simulink model "UAV_Task4_3"  (R2024b)
settings: Solver=ode45  StartTime=0  StopTime=100  RelTol=1e-5  AbsTol=1e-5
values from neighbouring files (symbols this model uses):
  adaptiveActivation = 1    [UAV_Task4_1_main.m]    (also in UAV_Task4_2_main.m = 0; UAV_Task4_3_main.m)
  B_p = 1/UAV.m    [UAV_Task4_1_main.m]    (also in UAV_Task4_2_main.m; UAV_Task4_3_main.m)
  F2plus = F2'*pinv(F2*F2')    [UAV_Task4_1_main.m]    (also in UAV_Task4_2_main.m; UAV_Task4_3_main.m)
  fe_0 = [0;0]    [UAV_Task4_3_main.m]
  Gamma_a = 1*[1 1 1 1]'    [UAV_Task4_1_main.m]    (also in UAV_Task4_2_main.m; UAV_Task4_3_main.m = 1*[1 1 1 1 1 1]')
  Gamma_a_scalar = 1    [UAV_Task4_2_main.m]    (also in UAV_Task4_3_main.m)
  gravityInAdaptiveController = 1    [UAV_Task4_1_main.m]    (also in UAV_Task4_2_main.m; UAV_Task4_3_main.m)
  k_f = 0.3379e-6    (= 3.379e-07)    [UAV_Task4_1_main.m]    (also in UAV_Task4_2_main.m; UAV_Task4_3_main.m)
  L = 10    [UAV_Task4_1_main.m]    (also in UAV_Task4_2_main.m; UAV_Task4_3_main.m)
  lambda_0 = 1    [UAV_Task4_1_main.m]    (also in UAV_Task4_2_main.m; UAV_Task4_3_main.m)
  Omega_0 = [1500 1500 1500 1500]'    [UAV_Task4_1_main.m]    (also in UAV_Task4_2_main.m; UAV_Task4_3_main.m)
  omegab_0 = [0; 0; 0]    [UAV_Task4_1_main.m]    (also in UAV_Task4_2_main.m; UAV_Task4_3_main.m)
  p_0 = [0; 0; 0]    [UAV_Task4_1_main.m]    (also in UAV_Task4_2_main.m; UAV_Task4_3_main.m)
  PO = 1    [UAV_Task4_1_main.m]    (also in UAV_Task4_2_main.m; UAV_Task4_3_main.m)
  q_0 = eul2quat([0, 0, 0]*degToRad,'ZYX')'    [UAV_Task4_1_main.m]    (also in UAV_Task4_2_main.m; UAV_Task4_3_main.m)
  scenario = 2    [UAV_Task4_1_main.m]    (also in UAV_Task4_2_main.m; UAV_Task4_3_main.m)
  theta_0 = [0.07;0.07;0.1]    [UAV_Task4_1_main.m]    (also in UAV_Task4_2_main.m; UAV_Task4_3_main.m)
  vb_0 = [0; 0; 0]    [UAV_Task4_1_main.m]    (also in UAV_Task4_2_main.m; UAV_Task4_3_main.m)
undefined symbols (not defined in the file or in its folder): adaptive_controller, ctrl, D_fv_i, dyn, e_3, epsilon_PO, fw_params_fc, g, lambda_i, par, pos, pos_pp, projection_operator, targetParams, theta_M, UAV, v_M, vel, vel_pp
libraries: slpidlib x22, matrix_library x6, aerolibutil x2, uavutilslib x1
(part 1 of 4)
settings Model: Creator=justs  LastModifiedBy=giuseppe
settings SolverCC: ZeroCrossAlgorithm=Adaptive
settings DataIOCC: SaveFormat=StructureWithTime
settings OptimizationCC: BlockReduction=off  BufferReuse=off  ReuseModelBlockBuffer=off
settings DebuggingCC: AlgebraicLoopMsg=none
settings ModelReferenceCC: EnableRefExpFcnMdlSchedulingChecks=on
settings RTWCC: GPUComputeCapability=3.5

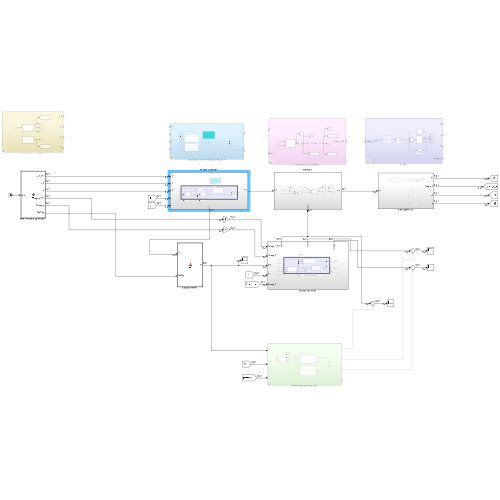
[thumbnail: Simulink's stored preview of the top-level diagram]
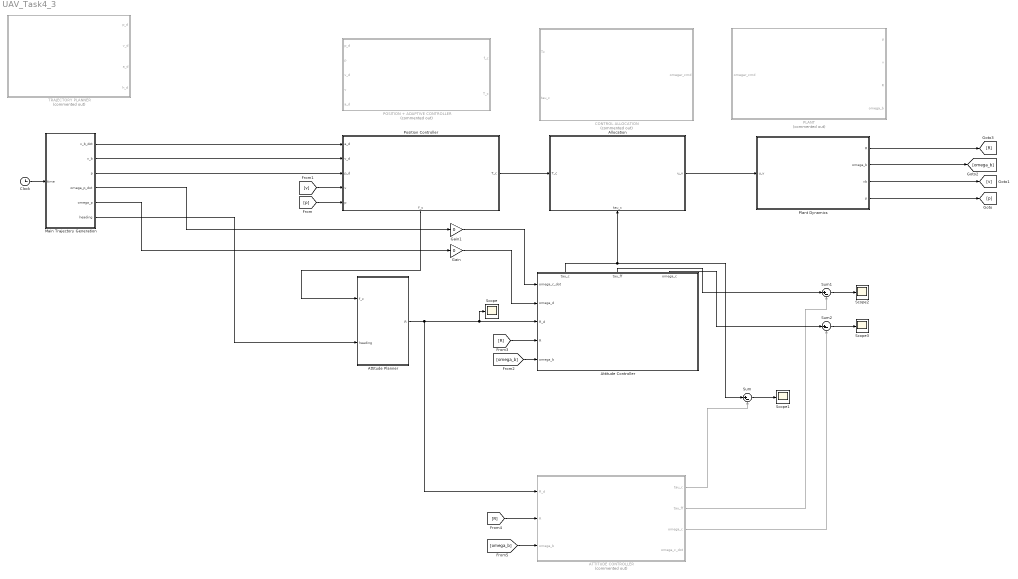
== system UAV_Task4_3 ==
  ATTITUDE CONTROLLER : Subsystem  Commented=on
  Allocation : Subsystem
      settings: PortSchema="{\"entries\":[{\"content\":{\"sides\":[{\"content\":{\"connectorIds\":[\"In1\"]},\"type\":\"ConnectorPlacement.EquallySpacedRectSide\",\"uuid\":\"a90dffa2-e17d-417b-aee2-5b49e390cc31\"},{\"content\":{\"connectorIds\":[\"Out1\"],\"side\":\"RIGHT\"},\"type\":\"ConnectorPlacement.EquallySpacedRectSide\",\"uuid\":\"68e70ff2-14f1-48b3-bfaa-1f22ab14f6ef\"},{\"content\":{\"side\":\"TOP\"},\"type\":\"ConnectorPlacement.EquallySpacedRectSide\",\"uuid\":\"a590dd5a-1e20-4e52-b823-4efe502fedb5\"},{\"content\":{\"connectorIds\":[\"In2\"],\"side\":\"BOTTOM\"},\"type\":\"ConnectorPlacement.EquallySpacedRectSide\",\"uuid\":\"c0eee0c2-1b4f-48e1-a09d-5bd9eaf490e9\"}]},\"type\":\"ConnectorPlacement.EquallySpacedConnector\",\"uuid\":\"29ee6c53-58dc-46de-8e17-ce1d472e0644\"}],\"packageUris\":[\"http://schema.mathworks.com/mf0/Connector/R2020b\"],\"version\":\"1.0\"}"
  Attitude Controller : Subsystem
      settings: PortSchema="{\"entries\":[{\"content\":{\"sides\":[{\"content\":{\"connectorIds\":[\"In1\",\"In2\",\"In3\",\"In4\",\"In5\"]},\"type\":\"ConnectorPlacement.EquallySpacedRectSide\",\"uuid\":\"fd474fdd-809e-484b-b672-45c162405a48\"},{\"content\":{\"side\":\"RIGHT\"},\"type\":\"ConnectorPlacement.EquallySpacedRectSide\",\"uuid\":\"9c86daaf-9aed-46d9-83bf-dcd411d29638\"},{\"content\":{\"connectorIds\":[\"Out1\",\"Out2\",\"Out3\"],\"side\":\"TOP\"},\"type\":\"ConnectorPlacement.EquallySpacedRectSide\",\"uuid\":\"8bdcf73f-78a3-4153-a3ad-0cecea352ffe\"}]},\"type\":\"ConnectorPlacement.EquallySpacedConnector\",\"uuid\":\"4a1693e7-34c2-4f2b-859c-49762a9733c3\"}],\"packageUris\":[\"http://schema.mathworks.com/mf0/Connector/R2020b\"],\"version\":\"1.0\"}"
  Attitude Planner : MATLAB Function  TreatAsAtomicUnit=on
  CONTROL ALLOCATION : Subsystem  Commented=on
  Clock : Clock
  Gain : Gain  Gain=0
  Gain1 : Gain  Gain=0
  Main Trajectory Generation : MATLAB Function  TreatAsAtomicUnit=on
  PLANT : Subsystem  Commented=on
  POSITION + ADAPTIVE CONTROLLER : Subsystem  Commented=on
  Plant Dynamics : Subsystem
  Position Controller : Subsystem
      settings: PortSchema="{\"entries\":[{\"content\":{\"sides\":[{\"content\":{\"connectorIds\":[\"In1\",\"In2\",\"In3\",\"In4\",\"In5\"]},\"type\":\"ConnectorPlacement.EquallySpacedRectSide\",\"uuid\":\"aaf371c6-7de6-4752-a94f-8f5eebff8076\"},{\"content\":{\"connectorIds\":[\"Out1\"],\"side\":\"RIGHT\"},\"type\":\"ConnectorPlacement.EquallySpacedRectSide\",\"uuid\":\"c91caa52-c2d3-4ced-bf24-c82d170a1382\"},{\"content\":{\"side\":\"TOP\"},\"type\":\"ConnectorPlacement.EquallySpacedRectSide\",\"uuid\":\"213f93cc-3232-43d4-924b-d32a630f7005\"},{\"content\":{\"connectorIds\":[\"Out2\"],\"side\":\"BOTTOM\"},\"type\":\"ConnectorPlacement.EquallySpacedRectSide\",\"uuid\":\"34712f80-774f-4a90-8ba5-2e5f701bc3fc\"}]},\"type\":\"ConnectorPlacement.EquallySpacedConnector\",\"uuid\":\"ff6af449-8110-47b4-88e9-388be9daf96b\"}],\"packageUris\":[\"http://schema.mathworks.com/mf0/Connector/R2020b\"],\"version\":\"1.0\"}"
  Scope{,1..3} (4 alike) : Scope
  Sum : Sum  Inputs=|+-
  Sum1 : Sum  Inputs=|+-
  Sum2 : Sum  Inputs=|+-
  TRAJECTORY PLANNER : Subsystem  Commented=on
  wires:
  Allocation/1(u_v) -> Plant Dynamics/1(u_v)
  Main Trajectory Generation/4(omega_p_dot) -> Gain1/1
  Main Trajectory Generation/5(omega_p) -> Gain/1
  Main Trajectory Generation/6(heading) -> Attitude Planner/2(heading)
  Position Controller/1(T_c) -> Allocation/1(T_c)
  [omega_b] -> Attitude Controller/5(omega_b)
  [R] -> Attitude Controller/4(R)
  Attitude Planner/1(R) -> ATTITUDE CONTROLLER/1(R_d), Attitude Controller/3(R_d), Scope/1
  Position Controller/2(f_c) -> Attitude Planner/1(f_c)
  [p] -> Position Controller/5(p)
  [v] -> Position Controller/4(v)
  Plant Dynamics/1(R) -> [R]
  Plant Dynamics/2(omega_b) -> [omega_b]
  Plant Dynamics/3(vb) -> [v]
  Plant Dynamics/4(p) -> [p]
  ATTITUDE CONTROLLER/1(tau_c) -> Sum/2
  Sum/1 -> Scope1/1
  Attitude Controller/1(tau_c) -> Allocation/2(tau_c), Sum/1
  [R] -> ATTITUDE CONTROLLER/2(R)
  [omega_b] -> ATTITUDE CONTROLLER/3(omega_b)
  Clock/1 -> Main Trajectory Generation/1(time)
  Main Trajectory Generation/3(p) -> Position Controller/3(p_d)
  Main Trajectory Generation/2(v_b) -> Position Controller/2(v_d)
  Main Trajectory Generation/1(v_b_dot) -> Position Controller/1(a_d)
  Sum1/1 -> Scope2/1
  Sum2/1 -> Scope3/1
  Attitude Controller/2(tau_ff) -> Sum1/1
  ATTITUDE CONTROLLER/2(tau_ff) -> Sum1/2
  ATTITUDE CONTROLLER/3(omega_c) -> Sum2/2
  Attitude Controller/3(omega_c) -> Sum2/1
  Gain/1 -> Attitude Controller/2(omega_d)
  Gain1/1 -> Attitude Controller/1(omega_c_dot)

== system UAV_Task4_3/ATTITUDE CONTROLLER ==
  R_d : Inport
  R : Inport  Port=2
  omega_b : Inport  Port=3
  Attitude dynamics FB : Subsystem
  Attitude dynamics FF : Subsystem
  Attitude kinematics : Subsystem
  Scope : Scope
  To Workspace : ToWorkspace  Commented=on  VariableName=tau_c  SaveFormat=Structure With Time  SampleTime=-1
  tau_c : Outport
  tau_ff : Outport  Port=2
  omega_c : Outport  Port=3
  omega_c_dot : Outport  Port=4
  wires:
  R_d/1 -> Attitude kinematics/1(R_d)
  Attitude kinematics/1(omega_c) -> omega_c/1, Scope/1, [omega_c]
  Attitude kinematics/2(omega_c_dot) -> omega_c_dot/1, [omega_c_dot]
  [omega_c] -> Attitude dynamics FF/1(omega_c)
  [omega_c_dot] -> Attitude dynamics FF/2(omega_c_dot)
  omega_b/1 -> Attitude dynamics FB/1(omega_b), Attitude dynamics FF/3(omega_b)
  R/1 -> Attitude kinematics/2(R)
  [omega_c] -> Attitude dynamics FB/2(omega_c)
  Attitude dynamics FF/1(tau_c) -> To Workspace/1, tau_c/1
  Attitude dynamics FF/2(tau_ff) -> tau_ff/1

== system UAV_Task4_3/Allocation ==
  T_c : Inport
  tau_c : Inport  Port=2
  Constant : Constant  Value=F2plus
  Matrix Multiply : Product  Multiplication=Matrix(*)
  Mux2 : Mux  Inputs=2
  Reshape : Reshape  OutputDimensionality=Column vector (2-D)
  Saturation : Saturate  Commented=through  UpperLimit=1000  LowerLimit=0
  Scope : Scope
  Scope1 : Scope
  Scope2 : Scope
  u_v : Outport
  wires:
  Mux2/1 -> Reshape/1
  tau_c/1 -> Mux2/2
  Reshape/1 -> Matrix Multiply/2
  Constant/1 -> Matrix Multiply/1
  Matrix Multiply/1 -> Scope1/1, Saturation/1  "u_v"
  T_c/1 -> Mux2/1, Scope/1
  Saturation/1 -> Scope2/1, u_v/1

== system UAV_Task4_3/Attitude Controller ==
  note: Attitude Controller
  omega_c_dot : Inport
  omega_d : Inport  Port=2
  R_d : Inport  Port=3
  R : Inport  Port=4
  omega_b : Inport  Port=5
  Attitude controller (Kin) : MATLAB Function  TreatAsAtomicUnit=on
  Attitude feedforward : MATLAB Function  TreatAsAtomicUnit=on
  Derivative : Derivative
  Feedback (Angular Velocity controller) (Dyn) : Subsystem
  Sum : Sum  Inputs=+-|
  Sum1 : Sum  Inputs=|-+
  To Workspace : ToWorkspace  VariableName=e_omega  SaveFormat=Timeseries  SampleTime=-1
  To Workspace1 : ToWorkspace  VariableName=tau_c  SaveFormat=Timeseries  SampleTime=-1
  To Workspace3 : ToWorkspace  VariableName=quat_e  SaveFormat=Timeseries  SampleTime=-1
  tau_c : Outport
  tau_ff : Outport  Port=2
  omega_c : Outport  Port=3
  wires:
  R/1 -> Attitude controller (Kin)/3(R)
  R_d/1 -> Attitude controller (Kin)/1(R_d)
  Attitude controller (Kin)/2(quat_e) -> To Workspace3/1
  Sum1/1 -> Feedback (Angular Velocity controller) (Dyn)/1(e_omega), To Workspace/1
  Feedback (Angular Velocity controller) (Dyn)/1(tau_fbk) -> Sum/2
  omega_b/1 -> Attitude feedforward/1(omega_b), Sum1/2
  omega_d/1 -> Attitude controller (Kin)/2(omega_d)
  Sum/1 -> tau_c/1, To Workspace1/1  "tau_c"
  Attitude feedforward/1(tau_ff) -> tau_ff/1, Sum/1
  Attitude controller (Kin)/1(omega_c) -> Derivative/1, omega_c/1, Attitude feedforward/3(omega_c), Sum1/1
  Derivative/1 -> Attitude feedforward/2(omega_c_dot)

== system UAV_Task4_3/CONTROL ALLOCATION ==
  Tc : Inport
  tau_c : Inport  Port=2
  Gain : Gain  Commented=through  Gain=1/k_f
  MATLAB Function1 : MATLAB Function  TreatAsAtomicUnit=on
  Saturation : Saturate  UpperLimit=3  LowerLimit=0.1
  Scope : Scope
  Scope1 : Scope
  Scope2 : Scope
  Sqrt : Sqrt  Commented=through
  To Workspace : ToWorkspace  VariableName=u_c  SaveFormat=Structure With Time  SampleTime=-1
  To Workspace1 : ToWorkspace  VariableName=omegar_cmd  SaveFormat=Timeseries  SampleTime=-1
  To Workspace2 : ToWorkspace  VariableName=omegar_cmd_array  SampleTime=-1
  omegar_cmd : Outport
  wires:
  Tc/1 -> MATLAB Function1/1(Tc)
  tau_c/1 -> MATLAB Function1/2(tau_c)
  Sqrt/1 -> To Workspace1/1, Scope2/1, To Workspace2/1, omegar_cmd/1
  MATLAB Function1/1(u_c) -> Saturation/1, Scope/1
  Saturation/1 -> Gain/1, Scope1/1, To Workspace/1
  Gain/1 -> Sqrt/1

== system UAV_Task4_3/PLANT ==
  note: w_g
  note: F*u
  note: Control wrench
  note: Damping wrench
  omegar_cmd : Inport
  Add : Sum  Inputs=++-
  Gain1 : Gain  Gain=UAV.F  Multiplication=Matrix(K*u)
  Gain2 : Gain  Gain=UAV.D  Multiplication=Matrix(K*u)
  Gravity wrench : MATLAB Function  TreatAsAtomicUnit=on
  Propeller dynamics : Subsystem  Commented=through
  "Rigid Body dynamics&kinematics " : Subsystem
  p : Outport
  v : Outport  Port=2
  R : Outport  Port=3
  omega_b : Outport  Port=4
  wires:
  "Rigid Body dynamics&kinematics "/5(nu_b) -> Gain2/1
  Gravity wrench/1(w_g) -> Add/1
  Add/1 -> "Rigid Body dynamics&kinematics "/1(w_b)
  "Rigid Body dynamics&kinematics "/2(R) -> Gravity wrench/1(R), R/1
  omegar_cmd/1 -> Propeller dynamics/1(omegar_cmd)
  Propeller dynamics/1(u) -> Gain1/1
  "Rigid Body dynamics&kinematics "/1(p) -> p/1
  Gain2/1 -> Add/3  "D*nu_b"
  "Rigid Body dynamics&kinematics "/4(omegab) -> omega_b/1
  "Rigid Body dynamics&kinematics "/3(vb) -> v/1
  Gain1/1 -> Add/2

== system UAV_Task4_3/POSITION + ADAPTIVE CONTROLLER ==
  p_d : Inport
  p : Inport  Port=2
  v_d : Inport  Port=3
  v : Inport  Port=4
  a_d : Inport  Port=5
  Constant1 : Constant  Value=adaptive_controller
  MATLAB Function : MATLAB Function  TreatAsAtomicUnit=on
  P/P PARALLEL CONTROLLER : Subsystem  Commented=on
  POSITION CONTROLLER : Subsystem
  Scope : Scope
  Scope1 : Scope
  Scope5 : Scope
  Subsystem1 : Subsystem
  Sum : Sum  Inputs=|+-
  Sum1 : Sum  Inputs=++|
  Switch1 : Switch  Criteria=u2 > Threshold  Threshold=0.5  SaturateOnIntegerOverflow=off  InputSameDT=off
  To Workspace : ToWorkspace  VariableName=f_c  SaveFormat=Structure With Time  SampleTime=-1
  To Workspace1 : ToWorkspace  VariableName=T_c  SaveFormat=Structure With Time  SampleTime=-1
  To Workspace2 : ToWorkspace  VariableName=p_error  SaveFormat=Timeseries  SampleTime=-1
  f_c : Outport
  T_c : Outport  Port=2
  wires:
  p_d/1 -> Sum/1, P/P PARALLEL CONTROLLER/1(p_d), POSITION CONTROLLER/1(p_d)
  p/1 -> Sum/2, P/P PARALLEL CONTROLLER/2(p), POSITION CONTROLLER/2(p)
  v_d/1 -> P/P PARALLEL CONTROLLER/3(v_d), POSITION CONTROLLER/3(v_d)
  v/1 -> Subsystem1/1(v), P/P PARALLEL CONTROLLER/4(v), POSITION CONTROLLER/4(v)
  MATLAB Function/1(T_c) -> To Workspace1/1, T_c/1
  Switch1/1 -> MATLAB Function/1(f_c), f_c/1, Scope/1, To Workspace/1
  Sum/1 -> Scope1/1, To Workspace2/1
  Sum1/1 -> Switch1/1, Scope5/1
  Constant1/1 -> Switch1/2
  POSITION CONTROLLER/1(f_c) -> Subsystem1/2(ub), Sum1/2, Switch1/3
  a_d/1 -> P/P PARALLEL CONTROLLER/5(a_d), POSITION CONTROLLER/5(a_d)
  Subsystem1/1(ua) -> Sum1/1

== system UAV_Task4_3/Plant Dynamics ==
  note: fix UAV.F and put it here
  note: Damping wrench
  note: F*u
  note: w_g
  u_v : Inport
  Add : Sum  Commented=on  Inputs=++-
  Attitude kinematics&dynamics : Subsystem
  Gain1 : Gain  Gain=UAV.F  Multiplication=Matrix(K*u)
  Gain2 : Gain  Commented=on  Gain=UAV.D  Multiplication=Matrix(K*u)
  Gravity wrench : MATLAB Function  Commented=on  TreatAsAtomicUnit=on
  "Rigid Body dynamics&kinematics " : Subsystem  Commented=on
  Rotor Dynamics : Subsystem
  R : Outport
  omega_b : Outport  Port=2
  vb : Outport  Port=3
  p : Outport  Port=4
  wires:
  u_v/1 -> Rotor Dynamics/1(T_cmd)
  Gain2/1 -> Add/3  "D*nu_b"
  "Rigid Body dynamics&kinematics "/5(nu_b) -> Gain2/1
  "Rigid Body dynamics&kinematics "/2(R) -> Gravity wrench/1(R)
  Gravity wrench/1(w_g) -> Add/1
  Add/1 -> "Rigid Body dynamics&kinematics "/1(w_b)
  Attitude kinematics&dynamics/1(p) -> p/1
  Attitude kinematics&dynamics/2(v_NED) -> vb/1
  Attitude kinematics&dynamics/3(omega_b) -> omega_b/1
  Attitude kinematics&dynamics/4(R) -> R/1
  Rotor Dynamics/1(Actual Thrust) -> Gain1/1
  Gain1/1 -> Attitude kinematics&dynamics/1(w_b)

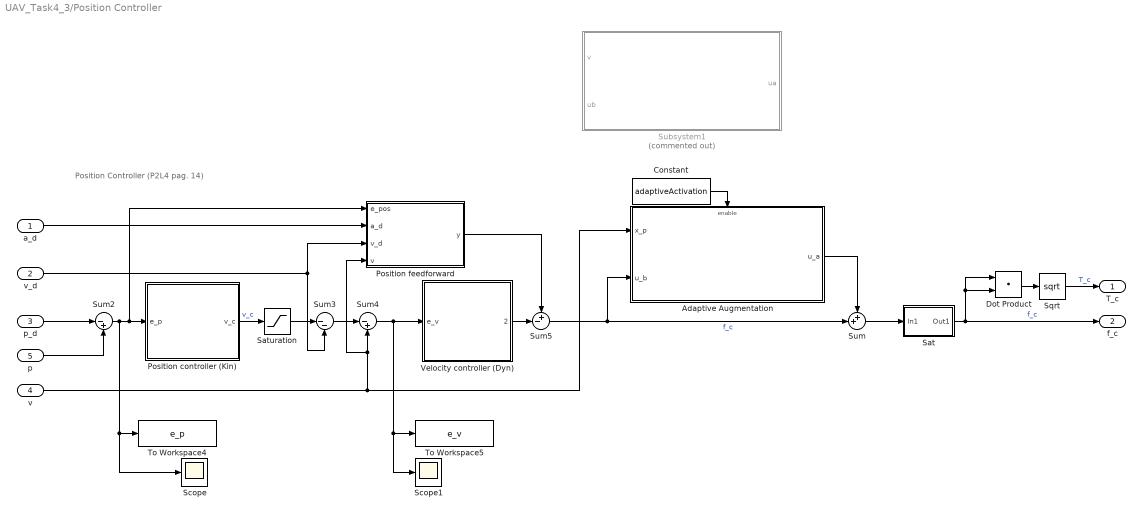
== system UAV_Task4_3/Position Controller ==
  note: Position Controller (P2L4 pag. 14)
  a_d : Inport
  v_d : Inport  Port=2
  p_d : Inport  Port=3
  v : Inport  Port=4
  p : Inport  Port=5
  Adaptive Augmentation : Subsystem
  Constant : Constant  Value=adaptiveActivation
  Dot Product : DotProduct  OutDataTypeStr=Inherit: Inherit via internal rule
  Position controller (Kin) : Subsystem
  Position feedforward : MATLAB Function  TreatAsAtomicUnit=on
  Sat : Subsystem
  Saturation : Saturate  UpperLimit=ctrl.vMax  LowerLimit=-ctrl.vMax
  Scope : Scope
  Scope1 : Scope
  Sqrt : Sqrt
  Subsystem1 : Subsystem  Commented=on
  Sum : Sum  Inputs=++|
  Sum2 : Sum  Inputs=|-+
  Sum3 : Sum  Inputs=|--
  Sum4 : Sum  Inputs=|-+
  Sum5 : Sum  Inputs=+-|
  To Workspace4 : ToWorkspace  VariableName=e_p  SaveFormat=Timeseries  SampleTime=-1
  To Workspace5 : ToWorkspace  VariableName=e_v  SaveFormat=Timeseries  SampleTime=-1
  Velocity controller (Dyn) : Subsystem
  T_c : Outport
  f_c : Outport  Port=2
  wires:
  p/1 -> Sum2/2
  a_d/1 -> Position feedforward/2(a_d)
  Sum4/1 -> Scope1/1, To Workspace5/1, Velocity controller (Dyn)/1(e_v)
  v_d/1 -> Sum3/2, Position feedforward/3(v_d)
  v/1 -> Adaptive Augmentation/1(x_p), Position feedforward/4(v), Sum4/2
  p_d/1 -> Sum2/1
  Velocity controller (Dyn)/1(2) -> Sum5/2
  Sum3/1 -> Sum4/1
  Sum2/1 -> Position feedforward/1(e_pos), Position controller (Kin)/1(e_p), Scope/1, To Workspace4/1
  Sum5/1 -> Adaptive Augmentation/2(u_b), Sum/2  "f_c"
  Position feedforward/1(y) -> Sum5/1
  Dot Product/1 -> Sqrt/1
  Sqrt/1 -> T_c/1  "T_c"
  Position controller (Kin)/1(v_c) -> Saturation/1  "v_c"
  Saturation/1 -> Sum3/1
  Sat/1(Out1) -> f_c/1, Dot Product/2, Dot Product/1  "f_c"
  Constant/1 -> Adaptive Augmentation/Enable
  Sum/1 -> Sat/1(In1)
  Adaptive Augmentation/1(u_a) -> Sum/1

== system UAV_Task4_3/TRAJECTORY PLANNER ==
  Clock : Clock
  Heading : MATLAB Function  TreatAsAtomicUnit=on
  To Workspace : ToWorkspace  VariableName=h_d  SaveFormat=Structure With Time  SampleTime=-1
  To Workspace1 : ToWorkspace  VariableName=p_d_array  SampleTime=-1
  Trajectory planner : MATLAB Function  TreatAsAtomicUnit=on
  p_d : Outport
  v_d : Outport  Port=2
  a_d : Outport  Port=3
  h_d : Outport  Port=4
  wires:
  Clock/1 -> Trajectory planner/1(t)
  Trajectory planner/3(a_d) -> a_d/1
  Trajectory planner/1(p_d) -> To Workspace1/1, p_d/1
  Trajectory planner/2(v_d) -> v_d/1
  Heading/1(h_d) -> h_d/1, To Workspace/1

== system UAV_Task4_3/ATTITUDE CONTROLLER/Attitude dynamics FB ==
  omega_b : Inport
  omega_c : Inport  Port=2
  Demux : Demux  Outputs=3
  Mux : Mux  Inputs=3
  PID Controller : slpidlib/PID Controller  Controller=PI  Form=Parallel  TimeDomain=Continuous-time  UseExternalTs=off  SampleTime=-1  IntegratorMethod=Forward Euler  FilterMethod=Forward Euler  ControllerParametersSource=internal  P=dyn.Kp(1,1)  I=dyn.Ki(1,1)  UseKiTs=off  D=dyn.Kd(1,1)  UseExternalDerivativeSource=off  N=100  UseFilter=on  TunerSelectOption=Transfer Function Based (PID Tuner App)  InitialConditionSource=internal  InitialConditionForIntegrator=0  InitialConditionForFilter=0  DifferentiatorICPrevScaledInput=0  ExternalReset=none  TrackingMode=off  Kt=1  LimitOutput=off  SatLimitsSource=internal  UpperSaturationLimit=inf  LowerSaturationLimit=-inf  LinearizeAsGain=on  AntiWindupMode=none  Kb=1  LimitIntegrator=off  UpperIntegratorSaturationLimit=inf  LowerIntegratorSaturationLimit=-inf  POutMin=[]  POutMax=[]  IOutMin=[]  IOutMax=[]  DOutMin=[]  DOutMax=[]  NOutMin=[]  NOutMax=[]  SumOutMin=[]  SumOutMax=[]  SaturationOutMin=[]  SaturationOutMax=[]  PParamMin=[]  PParamMax=[]  IParamMin=[]  IParamMax=[]  DParamMin=[]  DParamMax=[]  NParamMin=[]  NParamMax=[]  KbParamMin=[]  KbParamMax=[]  KtParamMin=[]  KtParamMax=[]  KbOutMin=[]  KbOutMax=[]  KtOutMin=[]  KtOutMax=[]  IntegratorOutMin=[]  IntegratorOutMax=[]  FilterOutMin=[]  FilterOutMax=[]  SumI1OutMin=[]  SumI1OutMax=[]  SumI2OutMin=[]  SumI2OutMax=[]  SumI3OutMin=[]  SumI3OutMax=[]  SumI4OutMin=[]  SumI4OutMax=[]  SumDOutMin=[]  SumDOutMax=[]  DifferentiatorOutMin=[]  DifferentiatorOutMax=[]  FilterDiffOutCoefMin=[]  FilterDiffOutCoefMax=[]  ReciprocalOutMin=[]  ReciprocalOutMax=[]  SumDenOutMin=[]  SumDenOutMax=[]  SumNumOutMin=[]  SumNumOutMax=[]  DivideOutMin=[]  DivideOutMax=[]  UdiffTsProdOutMin=[]  UdiffTsProdOutMax=[]  NTsProdOutMin=[]  NTsProdOutMax=[]  UintegralTsProdOutMin=[]  UintegralTsProdOutMax=[]  UngainTsProdOutMin=[]  UngainTsProdOutMax=[]  ClampingZeroOutDataTypeStr=Inherit: Inherit via back propagation  ClampingZeroOutMin=[]  ClampingZeroOutMax=[]  FilterDenConstantOutDataTypeStr=Inherit: Inherit via back propagation  FilterDenConstantOutMin=[]  FilterDenConstantOutMax=[]  PCopyOutDataTypeStr=Inherit: Inherit via back propagation  PCopyOutMin=[]  PCopyOutMax=[]  NCopyOutDataTypeStr=Inherit: Inherit via back propagation  NCopyOutMin=[]  NCopyOutMax=[]  IntegratorContinuousStateAttributes=''  IntegratorStateMustResolveToSignalObject=off  IntegratorRTWStateStorageClass=Auto  FilterContinuousStateAttributes=''  FilterStateMustResolveToSignalObject=off  FilterRTWStateStorageClass=Auto  ParallelPVariant=InternalParameters  IdealPVariant=Disabled  IVariant=InternalParameters  DVariant=Disabled  IntegratorVariant=Continuous  SatVariant=Disabled  AWVariant=Passthrough  PCopyVariant=Disabled  TRVariant=Disabled  FdbkBlocksVariant=Forward  IdealPFdbkVariant=Disabled  SatFdbkVariant=Disabled  DerivativeFilterVariant=Disabled  NVariant=Disabled  NCopyVariant=Disabled_SignalSpec  FilterICVariant=Disabled  IntegratorICVariant=InternalICs  ExternalResetVariant=Disabled  TRSumVariant=Passthrough  SumFdbkVariant=Disabled  SumVariant=Sum_PI  TsampFilterVariant=InternalTs  TsampNgainVariant=Passthrough  TsampIntegralVariant=Disabled_SignalSpec  ExternalSaturationOutDataTypeStr=Inherit: Same as second input  DerivativeSourceVariant=Disabled  PreIntVariant=InternalPreInt
  PID Controller1 : slpidlib/PID Controller  Controller=PI  Form=Parallel  TimeDomain=Continuous-time  UseExternalTs=off  SampleTime=-1  IntegratorMethod=Forward Euler  FilterMethod=Forward Euler  ControllerParametersSource=internal  P=dyn.Kp(2,2)  I=dyn.Ki(2,2)  UseKiTs=off  D=dyn.Kd(2,2)  UseExternalDerivativeSource=off  N=100  UseFilter=on  TunerSelectOption=Transfer Function Based (PID Tuner App)  InitialConditionSource=internal  InitialConditionForIntegrator=0  InitialConditionForFilter=0  DifferentiatorICPrevScaledInput=0  ExternalReset=none  TrackingMode=off  Kt=1  LimitOutput=off  SatLimitsSource=internal  UpperSaturationLimit=inf  LowerSaturationLimit=-inf  LinearizeAsGain=on  AntiWindupMode=none  Kb=1  LimitIntegrator=off  UpperIntegratorSaturationLimit=inf  LowerIntegratorSaturationLimit=-inf  POutMin=[]  POutMax=[]  IOutMin=[]  IOutMax=[]  DOutMin=[]  DOutMax=[]  NOutMin=[]  NOutMax=[]  SumOutMin=[]  SumOutMax=[]  SaturationOutMin=[]  SaturationOutMax=[]  PParamMin=[]  PParamMax=[]  IParamMin=[]  IParamMax=[]  DParamMin=[]  DParamMax=[]  NParamMin=[]  NParamMax=[]  KbParamMin=[]  KbParamMax=[]  KtParamMin=[]  KtParamMax=[]  KbOutMin=[]  KbOutMax=[]  KtOutMin=[]  KtOutMax=[]  IntegratorOutMin=[]  IntegratorOutMax=[]  FilterOutMin=[]  FilterOutMax=[]  SumI1OutMin=[]  SumI1OutMax=[]  SumI2OutMin=[]  SumI2OutMax=[]  SumI3OutMin=[]  SumI3OutMax=[]  SumI4OutMin=[]  SumI4OutMax=[]  SumDOutMin=[]  SumDOutMax=[]  DifferentiatorOutMin=[]  DifferentiatorOutMax=[]  FilterDiffOutCoefMin=[]  FilterDiffOutCoefMax=[]  ReciprocalOutMin=[]  ReciprocalOutMax=[]  SumDenOutMin=[]  SumDenOutMax=[]  SumNumOutMin=[]  SumNumOutMax=[]  DivideOutMin=[]  DivideOutMax=[]  UdiffTsProdOutMin=[]  UdiffTsProdOutMax=[]  NTsProdOutMin=[]  NTsProdOutMax=[]  UintegralTsProdOutMin=[]  UintegralTsProdOutMax=[]  UngainTsProdOutMin=[]  UngainTsProdOutMax=[]  ClampingZeroOutDataTypeStr=Inherit: Inherit via back propagation  ClampingZeroOutMin=[]  ClampingZeroOutMax=[]  FilterDenConstantOutDataTypeStr=Inherit: Inherit via back propagation  FilterDenConstantOutMin=[]  FilterDenConstantOutMax=[]  PCopyOutDataTypeStr=Inherit: Inherit via back propagation  PCopyOutMin=[]  PCopyOutMax=[]  NCopyOutDataTypeStr=Inherit: Inherit via back propagation  NCopyOutMin=[]  NCopyOutMax=[]  IntegratorContinuousStateAttributes=''  IntegratorStateMustResolveToSignalObject=off  IntegratorRTWStateStorageClass=Auto  FilterContinuousStateAttributes=''  FilterStateMustResolveToSignalObject=off  FilterRTWStateStorageClass=Auto  ParallelPVariant=InternalParameters  IdealPVariant=Disabled  IVariant=InternalParameters  DVariant=Disabled  IntegratorVariant=Continuous  SatVariant=Disabled  AWVariant=Passthrough  PCopyVariant=Disabled  TRVariant=Disabled  FdbkBlocksVariant=Forward  IdealPFdbkVariant=Disabled  SatFdbkVariant=Disabled  DerivativeFilterVariant=Disabled  NVariant=Disabled  NCopyVariant=Disabled_SignalSpec  FilterICVariant=Disabled  IntegratorICVariant=InternalICs  ExternalResetVariant=Disabled  TRSumVariant=Passthrough  SumFdbkVariant=Disabled  SumVariant=Sum_PI  TsampFilterVariant=InternalTs  TsampNgainVariant=Passthrough  TsampIntegralVariant=Disabled_SignalSpec  ExternalSaturationOutDataTypeStr=Inherit: Same as second input  DerivativeSourceVariant=Disabled  PreIntVariant=InternalPreInt
  PID Controller2 : slpidlib/PID Controller  Controller=PI  Form=Parallel  TimeDomain=Continuous-time  UseExternalTs=off  SampleTime=-1  IntegratorMethod=Forward Euler  FilterMethod=Forward Euler  ControllerParametersSource=internal  P=dyn.Kp(3,3)  I=dyn.Ki(3,3)  UseKiTs=off  D=dyn.Kd(3,3)  UseExternalDerivativeSource=off  N=100  UseFilter=on  TunerSelectOption=Transfer Function Based (PID Tuner App)  InitialConditionSource=internal  InitialConditionForIntegrator=0  InitialConditionForFilter=0  DifferentiatorICPrevScaledInput=0  ExternalReset=none  TrackingMode=off  Kt=1  LimitOutput=off  SatLimitsSource=internal  UpperSaturationLimit=inf  LowerSaturationLimit=-inf  LinearizeAsGain=on  AntiWindupMode=none  Kb=1  LimitIntegrator=off  UpperIntegratorSaturationLimit=inf  LowerIntegratorSaturationLimit=-inf  POutMin=[]  POutMax=[]  IOutMin=[]  IOutMax=[]  DOutMin=[]  DOutMax=[]  NOutMin=[]  NOutMax=[]  SumOutMin=[]  SumOutMax=[]  SaturationOutMin=[]  SaturationOutMax=[]  PParamMin=[]  PParamMax=[]  IParamMin=[]  IParamMax=[]  DParamMin=[]  DParamMax=[]  NParamMin=[]  NParamMax=[]  KbParamMin=[]  KbParamMax=[]  KtParamMin=[]  KtParamMax=[]  KbOutMin=[]  KbOutMax=[]  KtOutMin=[]  KtOutMax=[]  IntegratorOutMin=[]  IntegratorOutMax=[]  FilterOutMin=[]  FilterOutMax=[]  SumI1OutMin=[]  SumI1OutMax=[]  SumI2OutMin=[]  SumI2OutMax=[]  SumI3OutMin=[]  SumI3OutMax=[]  SumI4OutMin=[]  SumI4OutMax=[]  SumDOutMin=[]  SumDOutMax=[]  DifferentiatorOutMin=[]  DifferentiatorOutMax=[]  FilterDiffOutCoefMin=[]  FilterDiffOutCoefMax=[]  ReciprocalOutMin=[]  ReciprocalOutMax=[]  SumDenOutMin=[]  SumDenOutMax=[]  SumNumOutMin=[]  SumNumOutMax=[]  DivideOutMin=[]  DivideOutMax=[]  UdiffTsProdOutMin=[]  UdiffTsProdOutMax=[]  NTsProdOutMin=[]  NTsProdOutMax=[]  UintegralTsProdOutMin=[]  UintegralTsProdOutMax=[]  UngainTsProdOutMin=[]  UngainTsProdOutMax=[]  ClampingZeroOutDataTypeStr=Inherit: Inherit via back propagation  ClampingZeroOutMin=[]  ClampingZeroOutMax=[]  FilterDenConstantOutDataTypeStr=Inherit: Inherit via back propagation  FilterDenConstantOutMin=[]  FilterDenConstantOutMax=[]  PCopyOutDataTypeStr=Inherit: Inherit via back propagation  PCopyOutMin=[]  PCopyOutMax=[]  NCopyOutDataTypeStr=Inherit: Inherit via back propagation  NCopyOutMin=[]  NCopyOutMax=[]  IntegratorContinuousStateAttributes=''  IntegratorStateMustResolveToSignalObject=off  IntegratorRTWStateStorageClass=Auto  FilterContinuousStateAttributes=''  FilterStateMustResolveToSignalObject=off  FilterRTWStateStorageClass=Auto  ParallelPVariant=InternalParameters  IdealPVariant=Disabled  IVariant=InternalParameters  DVariant=Disabled  IntegratorVariant=Continuous  SatVariant=Disabled  AWVariant=Passthrough  PCopyVariant=Disabled  TRVariant=Disabled  FdbkBlocksVariant=Forward  IdealPFdbkVariant=Disabled  SatFdbkVariant=Disabled  DerivativeFilterVariant=Disabled  NVariant=Disabled  NCopyVariant=Disabled_SignalSpec  FilterICVariant=Disabled  IntegratorICVariant=InternalICs  ExternalResetVariant=Disabled  TRSumVariant=Passthrough  SumFdbkVariant=Disabled  SumVariant=Sum_PI  TsampFilterVariant=InternalTs  TsampNgainVariant=Passthrough  TsampIntegralVariant=Disabled_SignalSpec  ExternalSaturationOutDataTypeStr=Inherit: Same as second input  DerivativeSourceVariant=Disabled  PreIntVariant=InternalPreInt
  Scope : Scope
  Sum : Sum  Inputs=|+-
  tau_c : Outport
  wires:
  PID Controller2/1 -> Mux/3
  PID Controller/1 -> Mux/1
  Mux/1 -> tau_c/1
  Demux/3 -> PID Controller2/1
  omega_c/1 -> Sum/1
  Demux/1 -> PID Controller/1
  Sum/1 -> Scope/1, Demux/1
  PID Controller1/1 -> Mux/2
  Demux/2 -> PID Controller1/1
  omega_b/1 -> Sum/2

== system UAV_Task4_3/ATTITUDE CONTROLLER/Attitude dynamics FF ==
  omega_c : Inport
  omega_c_dot : Inport  Port=2
  omega_b : Inport  Port=3
  Feedback controller : Subsystem
  Scope2 : Scope
  Sum2 : Sum  Inputs=|++
  Sum3 : Sum  Inputs=|+-
  To Workspace2 : ToWorkspace  Commented=on  VariableName=e_omega  SaveFormat=Timeseries  SampleTime=-1
  feedforward : MATLAB Function  TreatAsAtomicUnit=on
  tau_c : Outport
  tau_ff : Outport  Port=2
  wires:
  omega_c_dot/1 -> feedforward/3(omega_c_dot)
  Sum3/1 -> To Workspace2/1, Feedback controller/1(e_omega)
  Sum2/1 -> tau_c/1
  omega_c/1 -> Sum3/1, feedforward/1(omega_c)
  feedforward/1(tau_ff) -> Scope2/1, tau_ff/1, Sum2/1
  Feedback controller/1(tau_fbk) -> Sum2/2
  omega_b/1 -> feedforward/2(omega_b), Sum3/2

== system UAV_Task4_3/ATTITUDE CONTROLLER/Attitude kinematics ==
  R_d : Inport
  R : Inport  Port=2
  Attitude controller P : MATLAB Function  TreatAsAtomicUnit=on
  Constant : Constant  Value=[0;0;0]
  Derivative2 : Derivative
  To Workspace6 : ToWorkspace  Commented=on  VariableName=quat_e  SaveFormat=Timeseries  SampleTime=-1
  omega_c : Outport
  omega_c_dot : Outport  Port=2
  wires:
  Attitude controller P/2(quat_e) -> To Workspace6/1
  Derivative2/1 -> omega_c_dot/1
  Attitude controller P/1(omega_c) -> omega_c/1, Derivative2/1
  R_d/1 -> Attitude controller P/2(R_d)
  R/1 -> Attitude controller P/1(R)
  Constant/1 -> Attitude controller P/3(omega_d)

== system UAV_Task4_3/Attitude Controller/Feedback (Angular Velocity controller) (Dyn) ==
  e_omega : Inport
  Demux : Demux  Outputs=3
  Mux : Mux  Inputs=3
  PID Controller p : slpidlib/PID Controller  Controller=PI  Form=Parallel  TimeDomain=Continuous-time  UseExternalTs=off  SampleTime=-1  IntegratorMethod=Forward Euler  FilterMethod=Forward Euler  ControllerParametersSource=internal  P=ctrl.Komega(1,1)  I=ctrl.Kiomega(1,1)  UseKiTs=off  D=0  UseExternalDerivativeSource=off  N=100  UseFilter=on  TunerSelectOption=Transfer Function Based (PID Tuner App)  InitialConditionSource=internal  InitialConditionForIntegrator=0  InitialConditionForFilter=0  DifferentiatorICPrevScaledInput=0  ExternalReset=none  TrackingMode=off  Kt=1  LimitOutput=off  SatLimitsSource=internal  UpperSaturationLimit=inf  LowerSaturationLimit=-inf  LinearizeAsGain=on  AntiWindupMode=none  Kb=1  LimitIntegrator=off  UpperIntegratorSaturationLimit=inf  LowerIntegratorSaturationLimit=-inf  POutMin=[]  POutMax=[]  IOutMin=[]  IOutMax=[]  DOutMin=[]  DOutMax=[]  NOutMin=[]  NOutMax=[]  SumOutMin=[]  SumOutMax=[]  SaturationOutMin=[]  SaturationOutMax=[]  PParamMin=[]  PParamMax=[]  IParamMin=[]  IParamMax=[]  DParamMin=[]  DParamMax=[]  NParamMin=[]  NParamMax=[]  KbParamMin=[]  KbParamMax=[]  KtParamMin=[]  KtParamMax=[]  KbOutMin=[]  KbOutMax=[]  KtOutMin=[]  KtOutMax=[]  IntegratorOutMin=[]  IntegratorOutMax=[]  FilterOutMin=[]  FilterOutMax=[]  SumI1OutMin=[]  SumI1OutMax=[]  SumI2OutMin=[]  SumI2OutMax=[]  SumI3OutMin=[]  SumI3OutMax=[]  SumI4OutMin=[]  SumI4OutMax=[]  SumDOutMin=[]  SumDOutMax=[]  DifferentiatorOutMin=[]  DifferentiatorOutMax=[]  FilterDiffOutCoefMin=[]  FilterDiffOutCoefMax=[]  ReciprocalOutMin=[]  ReciprocalOutMax=[]  SumDenOutMin=[]  SumDenOutMax=[]  SumNumOutMin=[]  SumNumOutMax=[]  DivideOutMin=[]  DivideOutMax=[]  UdiffTsProdOutMin=[]  UdiffTsProdOutMax=[]  NTsProdOutMin=[]  NTsProdOutMax=[]  UintegralTsProdOutMin=[]  UintegralTsProdOutMax=[]  UngainTsProdOutMin=[]  UngainTsProdOutMax=[]  ClampingZeroOutDataTypeStr=Inherit: Inherit via back propagation  ClampingZeroOutMin=[]  ClampingZeroOutMax=[]  FilterDenConstantOutDataTypeStr=Inherit: Inherit via back propagation  FilterDenConstantOutMin=[]  FilterDenConstantOutMax=[]  PCopyOutDataTypeStr=Inherit: Inherit via back propagation  PCopyOutMin=[]  PCopyOutMax=[]  NCopyOutDataTypeStr=Inherit: Inherit via back propagation  NCopyOutMin=[]  NCopyOutMax=[]  IntegratorContinuousStateAttributes=''  IntegratorStateMustResolveToSignalObject=off  IntegratorRTWStateStorageClass=Auto  FilterContinuousStateAttributes=''  FilterStateMustResolveToSignalObject=off  FilterRTWStateStorageClass=Auto  ParallelPVariant=InternalParameters  IdealPVariant=Disabled  IVariant=InternalParameters  DVariant=Disabled  IntegratorVariant=Continuous  SatVariant=Disabled  AWVariant=Passthrough  PCopyVariant=Disabled  TRVariant=Disabled  FdbkBlocksVariant=Forward  IdealPFdbkVariant=Disabled  SatFdbkVariant=Disabled  DerivativeFilterVariant=Disabled  NVariant=Disabled  NCopyVariant=Disabled_SignalSpec  FilterICVariant=Disabled  IntegratorICVariant=InternalICs  ExternalResetVariant=Disabled  TRSumVariant=Passthrough  SumFdbkVariant=Disabled  SumVariant=Sum_PI  TsampFilterVariant=InternalTs  TsampNgainVariant=Passthrough  TsampIntegralVariant=Disabled_SignalSpec  ExternalSaturationOutDataTypeStr=Inherit: Same as second input  DerivativeSourceVariant=Disabled  PreIntVariant=InternalPreInt
  PID Controller q : slpidlib/PID Controller  Controller=PI  Form=Parallel  TimeDomain=Continuous-time  UseExternalTs=off  SampleTime=-1  IntegratorMethod=Forward Euler  FilterMethod=Forward Euler  ControllerParametersSource=internal  P=ctrl.Komega(2,2)  I=ctrl.Kiomega(2,2)  UseKiTs=off  D=0  UseExternalDerivativeSource=off  N=100  UseFilter=on  TunerSelectOption=Transfer Function Based (PID Tuner App)  InitialConditionSource=internal  InitialConditionForIntegrator=0  InitialConditionForFilter=0  DifferentiatorICPrevScaledInput=0  ExternalReset=none  TrackingMode=off  Kt=1  LimitOutput=off  SatLimitsSource=internal  UpperSaturationLimit=inf  LowerSaturationLimit=-inf  LinearizeAsGain=on  AntiWindupMode=none  Kb=1  LimitIntegrator=off  UpperIntegratorSaturationLimit=inf  LowerIntegratorSaturationLimit=-inf  POutMin=[]  POutMax=[]  IOutMin=[]  IOutMax=[]  DOutMin=[]  DOutMax=[]  NOutMin=[]  NOutMax=[]  SumOutMin=[]  SumOutMax=[]  SaturationOutMin=[]  SaturationOutMax=[]  PParamMin=[]  PParamMax=[]  IParamMin=[]  IParamMax=[]  DParamMin=[]  DParamMax=[]  NParamMin=[]  NParamMax=[]  KbParamMin=[]  KbParamMax=[]  KtParamMin=[]  KtParamMax=[]  KbOutMin=[]  KbOutMax=[]  KtOutMin=[]  KtOutMax=[]  IntegratorOutMin=[]  IntegratorOutMax=[]  FilterOutMin=[]  FilterOutMax=[]  SumI1OutMin=[]  SumI1OutMax=[]  SumI2OutMin=[]  SumI2OutMax=[]  SumI3OutMin=[]  SumI3OutMax=[]  SumI4OutMin=[]  SumI4OutMax=[]  SumDOutMin=[]  SumDOutMax=[]  DifferentiatorOutMin=[]  DifferentiatorOutMax=[]  FilterDiffOutCoefMin=[]  FilterDiffOutCoefMax=[]  ReciprocalOutMin=[]  ReciprocalOutMax=[]  SumDenOutMin=[]  SumDenOutMax=[]  SumNumOutMin=[]  SumNumOutMax=[]  DivideOutMin=[]  DivideOutMax=[]  UdiffTsProdOutMin=[]  UdiffTsProdOutMax=[]  NTsProdOutMin=[]  NTsProdOutMax=[]  UintegralTsProdOutMin=[]  UintegralTsProdOutMax=[]  UngainTsProdOutMin=[]  UngainTsProdOutMax=[]  ClampingZeroOutDataTypeStr=Inherit: Inherit via back propagation  ClampingZeroOutMin=[]  ClampingZeroOutMax=[]  FilterDenConstantOutDataTypeStr=Inherit: Inherit via back propagation  FilterDenConstantOutMin=[]  FilterDenConstantOutMax=[]  PCopyOutDataTypeStr=Inherit: Inherit via back propagation  PCopyOutMin=[]  PCopyOutMax=[]  NCopyOutDataTypeStr=Inherit: Inherit via back propagation  NCopyOutMin=[]  NCopyOutMax=[]  IntegratorContinuousStateAttributes=''  IntegratorStateMustResolveToSignalObject=off  IntegratorRTWStateStorageClass=Auto  FilterContinuousStateAttributes=''  FilterStateMustResolveToSignalObject=off  FilterRTWStateStorageClass=Auto  ParallelPVariant=InternalParameters  IdealPVariant=Disabled  IVariant=InternalParameters  DVariant=Disabled  IntegratorVariant=Continuous  SatVariant=Disabled  AWVariant=Passthrough  PCopyVariant=Disabled  TRVariant=Disabled  FdbkBlocksVariant=Forward  IdealPFdbkVariant=Disabled  SatFdbkVariant=Disabled  DerivativeFilterVariant=Disabled  NVariant=Disabled  NCopyVariant=Disabled_SignalSpec  FilterICVariant=Disabled  IntegratorICVariant=InternalICs  ExternalResetVariant=Disabled  TRSumVariant=Passthrough  SumFdbkVariant=Disabled  SumVariant=Sum_PI  TsampFilterVariant=InternalTs  TsampNgainVariant=Passthrough  TsampIntegralVariant=Disabled_SignalSpec  ExternalSaturationOutDataTypeStr=Inherit: Same as second input  DerivativeSourceVariant=Disabled  PreIntVariant=InternalPreInt
  PID Controller r : slpidlib/PID Controller  Controller=PI  Form=Parallel  TimeDomain=Continuous-time  UseExternalTs=off  SampleTime=-1  IntegratorMethod=Forward Euler  FilterMethod=Forward Euler  ControllerParametersSource=internal  P=ctrl.Komega(3,3)  I=ctrl.Kiomega(3,3)  UseKiTs=off  D=0  UseExternalDerivativeSource=off  N=100  UseFilter=on  TunerSelectOption=Transfer Function Based (PID Tuner App)  InitialConditionSource=internal  InitialConditionForIntegrator=0  InitialConditionForFilter=0  DifferentiatorICPrevScaledInput=0  ExternalReset=none  TrackingMode=off  Kt=1  LimitOutput=off  SatLimitsSource=internal  UpperSaturationLimit=inf  LowerSaturationLimit=-inf  LinearizeAsGain=on  AntiWindupMode=none  Kb=1  LimitIntegrator=off  UpperIntegratorSaturationLimit=inf  LowerIntegratorSaturationLimit=-inf  POutMin=[]  POutMax=[]  IOutMin=[]  IOutMax=[]  DOutMin=[]  DOutMax=[]  NOutMin=[]  NOutMax=[]  SumOutMin=[]  SumOutMax=[]  SaturationOutMin=[]  SaturationOutMax=[]  PParamMin=[]  PParamMax=[]  IParamMin=[]  IParamMax=[]  DParamMin=[]  DParamMax=[]  NParamMin=[]  NParamMax=[]  KbParamMin=[]  KbParamMax=[]  KtParamMin=[]  KtParamMax=[]  KbOutMin=[]  KbOutMax=[]  KtOutMin=[]  KtOutMax=[]  IntegratorOutMin=[]  IntegratorOutMax=[]  FilterOutMin=[]  FilterOutMax=[]  SumI1OutMin=[]  SumI1OutMax=[]  SumI2OutMin=[]  SumI2OutMax=[]  SumI3OutMin=[]  SumI3OutMax=[]  SumI4OutMin=[]  SumI4OutMax=[]  SumDOutMin=[]  SumDOutMax=[]  DifferentiatorOutMin=[]  DifferentiatorOutMax=[]  FilterDiffOutCoefMin=[]  FilterDiffOutCoefMax=[]  ReciprocalOutMin=[]  ReciprocalOutMax=[]  SumDenOutMin=[]  SumDenOutMax=[]  SumNumOutMin=[]  SumNumOutMax=[]  DivideOutMin=[]  DivideOutMax=[]  UdiffTsProdOutMin=[]  UdiffTsProdOutMax=[]  NTsProdOutMin=[]  NTsProdOutMax=[]  UintegralTsProdOutMin=[]  UintegralTsProdOutMax=[]  UngainTsProdOutMin=[]  UngainTsProdOutMax=[]  ClampingZeroOutDataTypeStr=Inherit: Inherit via back propagation  ClampingZeroOutMin=[]  ClampingZeroOutMax=[]  FilterDenConstantOutDataTypeStr=Inherit: Inherit via back propagation  FilterDenConstantOutMin=[]  FilterDenConstantOutMax=[]  PCopyOutDataTypeStr=Inherit: Inherit via back propagation  PCopyOutMin=[]  PCopyOutMax=[]  NCopyOutDataTypeStr=Inherit: Inherit via back propagation  NCopyOutMin=[]  NCopyOutMax=[]  IntegratorContinuousStateAttributes=''  IntegratorStateMustResolveToSignalObject=off  IntegratorRTWStateStorageClass=Auto  FilterContinuousStateAttributes=''  FilterStateMustResolveToSignalObject=off  FilterRTWStateStorageClass=Auto  ParallelPVariant=InternalParameters  IdealPVariant=Disabled  IVariant=InternalParameters  DVariant=Disabled  IntegratorVariant=Continuous  SatVariant=Disabled  AWVariant=Passthrough  PCopyVariant=Disabled  TRVariant=Disabled  FdbkBlocksVariant=Forward  IdealPFdbkVariant=Disabled  SatFdbkVariant=Disabled  DerivativeFilterVariant=Disabled  NVariant=Disabled  NCopyVariant=Disabled_SignalSpec  FilterICVariant=Disabled  IntegratorICVariant=InternalICs  ExternalResetVariant=Disabled  TRSumVariant=Passthrough  SumFdbkVariant=Disabled  SumVariant=Sum_PI  TsampFilterVariant=InternalTs  TsampNgainVariant=Passthrough  TsampIntegralVariant=Disabled_SignalSpec  ExternalSaturationOutDataTypeStr=Inherit: Same as second input  DerivativeSourceVariant=Disabled  PreIntVariant=InternalPreInt
  tau_fbk : Outport
  wires:
  PID Controller q/1 -> Mux/2
  Demux/2 -> PID Controller q/1
  e_omega/1 -> Demux/1
  Demux/3 -> PID Controller r/1
  PID Controller p/1 -> Mux/1
  PID Controller r/1 -> Mux/3
  Demux/1 -> PID Controller p/1
  Mux/1 -> tau_fbk/1

== system UAV_Task4_3/PLANT/Propeller dynamics ==
  note: PROPELLER DYNAMICS
  omegar_cmd : Inport
  Gain : Gain  Gain=k_f
  Gain1 : Gain  Gain=-UAV.k_m
  Gain2 : Gain  Gain=sqrt(UAV.lambda_r)  Multiplication=Matrix(K*u)
  Integrator : Integrator  InitialCondition=Omega_0
  Saturation : Saturate  UpperLimit=UAV.T_max  LowerLimit=UAV.T_min
  Square : Math  Operator=square
  Sum : Sum  Inputs=|+-
  To Workspace : ToWorkspace  VariableName=u  SaveFormat=Structure With Time  SampleTime=-1
  u : Outport
  wires:
  Gain1/1 -> Integrator/1  "omegar_dot"
  Integrator/1 -> Sum/1, Square/1  "omegar"
  Square/1 -> Gain/1
  Gain2/1 -> Sum/2
  omegar_cmd/1 -> Gain2/1
  Sum/1 -> Gain1/1
  Gain/1 -> Saturation/1
  Saturation/1 -> To Workspace/1, u/1

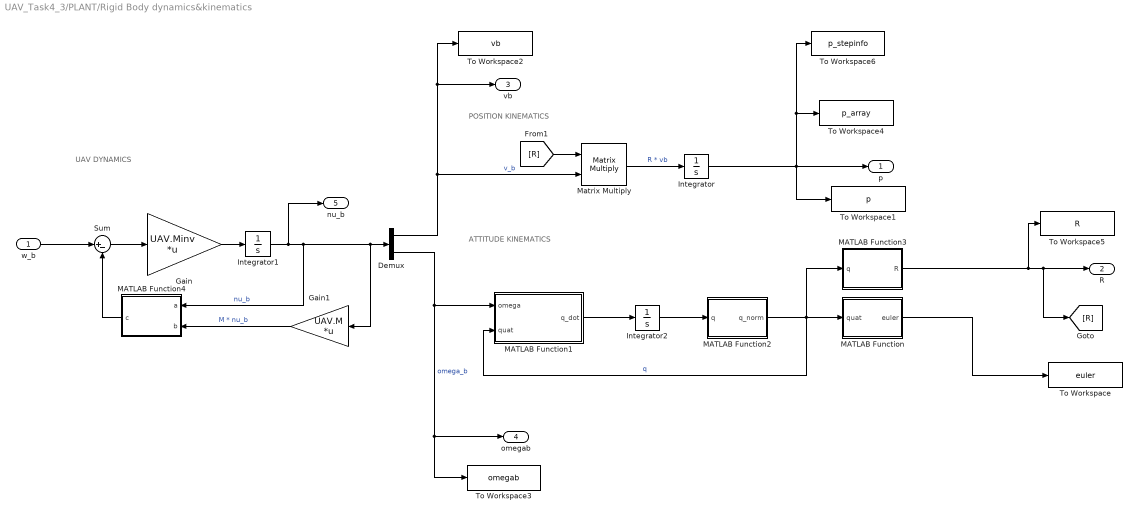
== system UAV_Task4_3/PLANT/Rigid Body dynamics&kinematics  ==
  note: UAV DYNAMICS
  note: ATTITUDE KINEMATICS
  note: POSITION KINEMATICS
  w_b : Inport
  Demux : Demux  Outputs=2
  Gain : Gain  Gain=UAV.Minv  Multiplication=Matrix(K*u)
  Gain1 : Gain  Gain=UAV.M  Multiplication=Matrix(K*u)
  Integrator : Integrator  InitialCondition=p_0
  Integrator1 : Integrator  InitialCondition=[vb_0;omegab_0]
  Integrator2 : Integrator  InitialCondition=q_0
  MATLAB Function : MATLAB Function  TreatAsAtomicUnit=on
  MATLAB Function1 : MATLAB Function  TreatAsAtomicUnit=on
  MATLAB Function2 : MATLAB Function  TreatAsAtomicUnit=on
  MATLAB Function3 : MATLAB Function  TreatAsAtomicUnit=on
  MATLAB Function4 : MATLAB Function  TreatAsAtomicUnit=on
  Matrix Multiply : Product  Multiplication=Matrix(*)
  Sum : Sum  Inputs=|+-
  To Workspace : ToWorkspace  VariableName=euler  SaveFormat=Timeseries  SampleTime=-1
  To Workspace1 : ToWorkspace  VariableName=p  SaveFormat=Timeseries  SampleTime=-1
  To Workspace2 : ToWorkspace  VariableName=vb  SaveFormat=Timeseries  SampleTime=-1
  To Workspace3 : ToWorkspace  VariableName=omegab  SaveFormat=Timeseries  SampleTime=-1
  To Workspace4 : ToWorkspace  VariableName=p_array  SampleTime=-1
  To Workspace5 : ToWorkspace  VariableName=R  SaveFormat=Structure With Time  SampleTime=-1
  To Workspace6 : ToWorkspace  VariableName=p_stepinfo  SaveFormat=Structure With Time  SampleTime=-1
  p : Outport
  R : Outport  Port=2
  vb : Outport  Port=3
  omegab : Outport  Port=4
  nu_b : Outport  Port=5
  wires:
  Integrator/1 -> To Workspace6/1, To Workspace4/1, p/1, To Workspace1/1
  MATLAB Function1/1(q_dot) -> Integrator2/1
  MATLAB Function2/1(q_norm) -> MATLAB Function3/1(q), MATLAB Function1/2(quat), MATLAB Function/1(quat)  "q"
  MATLAB Function3/1(R) -> R/1, [R], To Workspace5/1
  Demux/1 -> vb/1, To Workspace2/1, Matrix Multiply/2  "v_b"
  Integrator1/1 -> nu_b/1, Demux/1, Gain1/1, MATLAB Function4/1(a)  "nu_b"
  Integrator2/1 -> MATLAB Function2/1(q)
  Matrix Multiply/1 -> Integrator/1  "R * vb"
  MATLAB Function/1(euler) -> To Workspace/1
  [R] -> Matrix Multiply/1
  Gain/1 -> Integrator1/1
  Demux/2 -> omegab/1, To Workspace3/1, MATLAB Function1/1(omega)  "omega_b"
  Gain1/1 -> MATLAB Function4/2(b)  "M * nu_b"
  Sum/1 -> Gain/1
  MATLAB Function4/1(c) -> Sum/2
  w_b/1 -> Sum/1
